simulink model "PAlab3_2_4"  (R2025a)
settings: Solver=VariableStepAuto  StartTime=0.0  StopTime=10.0  RelTol=1e-3
settings Model: Creator=mieszko  LastModifiedBy=mieszko

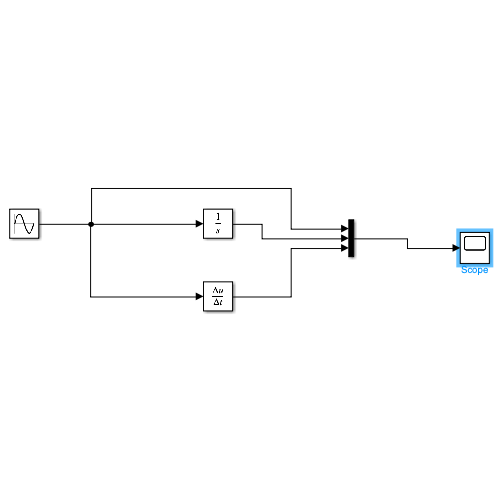
[thumbnail: Simulink's stored preview of the top-level diagram]
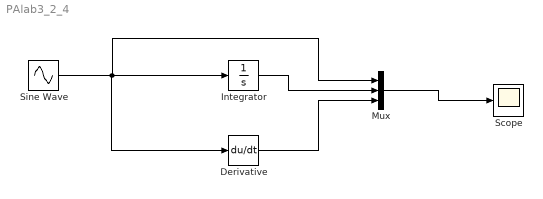
== system PAlab3_2_4 ==
  Derivative : Derivative
  Integrator : Integrator
  Mux : Mux  Inputs=3
  Scope : Scope
      settings: ActiveDisplayYMinimum=-1.3721162323558234  ActiveDisplayYMaximum=2.3743385168300524
  Sine Wave : Sin  SampleTime=0
  wires:
  Mux/1 -> Scope/1
  Integrator/1 -> Mux/2
  Derivative/1 -> Mux/3
  Sine Wave/1 -> Derivative/1, Mux/1, Integrator/1
